simulink model "task_4_sim"  (R2023a)
settings: Solver=VariableStepAuto  StartTime=0.0  StopTime=10.0  RelTol=1e-8
undefined symbols (not defined in the file): A, B, C, D, G, K, Q, x0, Y, z0
settings Model: Creator=user  LastModifiedBy=user

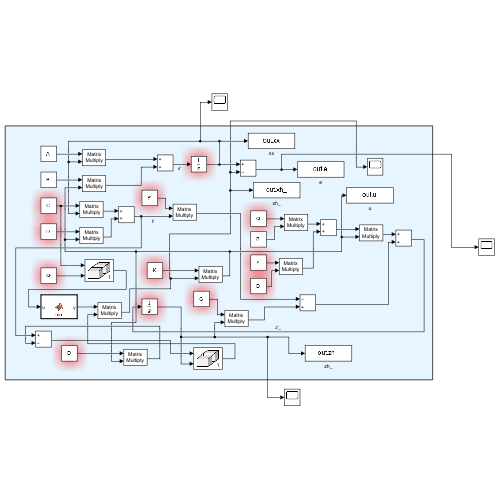
[thumbnail: Simulink's stored preview of the top-level diagram]
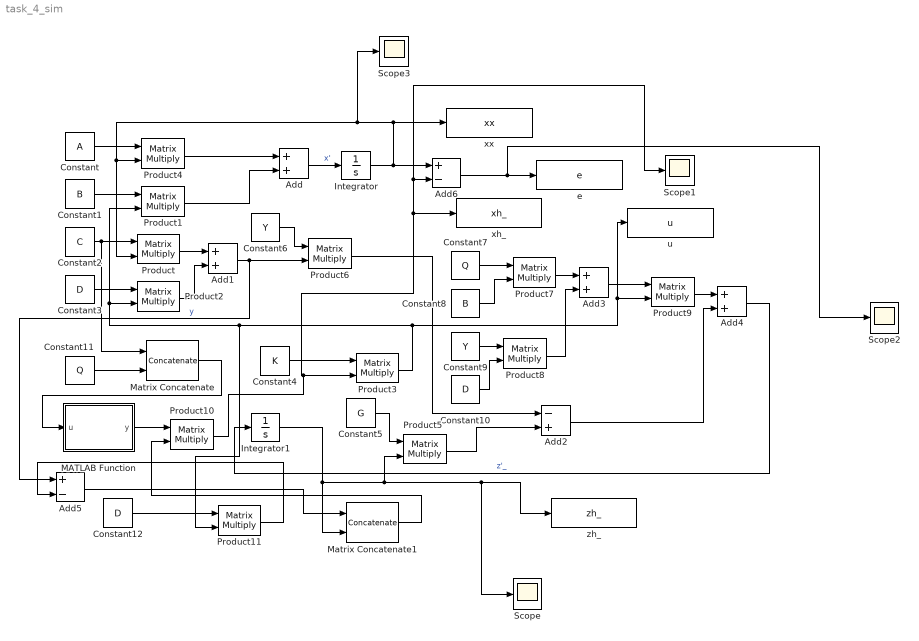
== system task_4_sim ==
  Add{,1,3..4} (4 alike) : Sum
  Add2 : Sum  Inputs=-+
  Add5 : Sum  Inputs=+-
  Add6 : Sum  Inputs=+-
  Constant : Constant  Value=A  VectorParams1D=off
  Constant1 : Constant  Value=B  VectorParams1D=off
  Constant10 : Constant  Value=D  VectorParams1D=off
  Constant11 : Constant  Value=Q  VectorParams1D=off
  Constant12 : Constant  Value=D  VectorParams1D=off
  Constant2 : Constant  Value=C  VectorParams1D=off
  Constant3 : Constant  Value=D  VectorParams1D=off
  Constant4 : Constant  Value=K  VectorParams1D=off
  Constant5 : Constant  Value=G  VectorParams1D=off
  Constant6 : Constant  Value=Y  VectorParams1D=off
  Constant7 : Constant  Value=Q  VectorParams1D=off
  Constant8 : Constant  Value=B  VectorParams1D=off
  Constant9 : Constant  Value=Y  VectorParams1D=off
  Integrator : Integrator  InitialCondition=x0
  Integrator1 : Integrator  InitialCondition=z0
  MATLAB Function : MATLAB Function  TreatAsAtomicUnit=on
  Matrix Concatenate : Concatenate  Mode=Multidimensional array
  Matrix Concatenate1 : Concatenate  Mode=Multidimensional array
  Product{,1..11} (12 alike) : Product  Multiplication=Matrix(*)
  Scope{,1..3} (4 alike) : Scope
  e : ToWorkspace  VariableName=e  SaveFormat=Timeseries  SampleTime=-1
  u : ToWorkspace  VariableName=u  SaveFormat=Timeseries  SampleTime=-1
  xh_ : ToWorkspace  VariableName=xh_  SaveFormat=Timeseries  SampleTime=-1
  xx : ToWorkspace  VariableName=xx  SaveFormat=Timeseries  SampleTime=-1
  zh_ : ToWorkspace  VariableName=zh_  SaveFormat=Timeseries  SampleTime=-1
  wires:
  Constant/1 -> Product4/1
  Integrator/1 -> Add6/1, Scope3/1, Product4/2, Product/2, xx/1
  Product4/1 -> Add/1
  Add/1 -> Integrator/1  "x'"
  Constant1/1 -> Product1/1
  Product1/1 -> Add/2
  Constant2/1 -> Matrix Concatenate/1, Product/1
  Constant3/1 -> Product2/1
  Product/1 -> Add1/1
  Product2/1 -> Add1/2
  Add1/1 -> Add5/1, Product6/2  "y"
  Constant4/1 -> Product3/1
  Product3/1 -> Product2/2, Product1/2, Product11/2, u/1, Product9/2
  Product10/1 -> Scope1/1, Add6/2, xh_/1, Product3/2
  Integrator1/1 -> Matrix Concatenate1/2, Scope/1, zh_/1, Product5/2
  Constant5/1 -> Product5/1
  Constant6/1 -> Product6/1
  Product6/1 -> Add2/1
  Product5/1 -> Add2/2
  Add2/1 -> Add4/2
  Constant7/1 -> Product7/1
  Constant8/1 -> Product7/2
  Constant9/1 -> Product8/1
  Constant10/1 -> Product8/2
  Product7/1 -> Add3/1
  Product8/1 -> Add3/2
  Add3/1 -> Product9/1
  Product9/1 -> Add4/1
  Add4/1 -> Integrator1/1  "z'_"
  Constant11/1 -> Matrix Concatenate/2
  Matrix Concatenate/1 -> MATLAB Function/1(u)
  MATLAB Function/1(y) -> Product10/1
  Constant12/1 -> Product11/1
  Product11/1 -> Add5/2
  Add5/1 -> Matrix Concatenate1/1
  Matrix Concatenate1/1 -> Product10/2
  Add6/1 -> Scope2/1, e/1

== matlab function task_4_sim/MATLAB Function ==
  data: u input; y output
function y = fcn(u)
y = pinv(u);
end
